simulink model "PatientModelCL"  (R2018a)
settings: Solver=VariableStepAuto  StartTime=0.0  StopTime=60*24  FixedStep=0.1  MaxStep=1
model workspace (MAT data in the model file):
  C = tf
  C.IOSize_ = [1 1]
  C.Data_ = ltipack.tfdata
  C.Data_.num = {[-7.005 -0.50005 -0.005]}
  C.Data_.den = {[0.01 1 0]}
  C.Data_.Delay.Input = 0
  C.Data_.Delay.Output = 0
  C.Data_.Delay.IO = 0
  C.Data_.Ts = 0
  params = Simulink.Parameter
  params.Value = [95.3858788985 10.0271565757 0.00997687337637 134.373440816 0.198499579953 0.00617711726591 0 13.4106496891 95.4135393331 143.03636756 131.139933532 0 0 0 0 0 0 0 0 0]
  params.DataType = 'auto'
  params.Dimensions = [1 20]
values from neighbouring files (symbols this model uses):
  params = mdlWks.getVariable('params')    [closedLoopSim.m]    (also in openLoopSim.m)
libraries: cstblocks x1
settings Model: OrderedModelArguments=off  Creator=vjoukov  LastModifiedBy=ms2wilso
settings SolverCC: InitialStep=.001
settings DataIOCC: ExternalInput=inputStruct  LoadExternalInput=on
settings ModelReferenceCC: ModelReferenceMinAlgLoopOccurrences=on

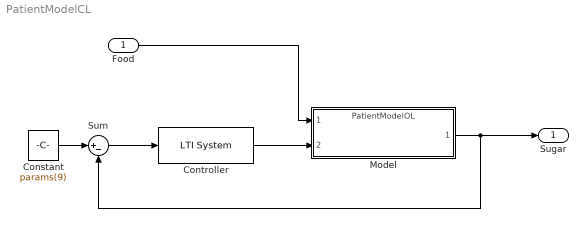
== system PatientModelCL ==
  Food : Inport
  Constant : Constant  Value=params(9)
  Controller : cstblocks/LTI System  sys=C  IC=[]
  Model : ModelReference  ModelNameDialog=PatientModelOL.slxp  ParameterArgumentNames=params  ParameterArgumentValues=params  UsingDefaultArgumentValue=0  ModelReferenceVersion=1.386  CopyOfModelProtected=on
  Sum : Sum  Inputs=|+-
  Sugar : Outport
  wires:
  Food/1 -> Model/1
  Model/1 -> Sum/2, Sugar/1
  Controller/1 -> Model/2
  Sum/1 -> Controller/1
  Constant/1 -> Sum/1
